simulink model "distortion_v4_1_saturation"  (R2018b)
settings: Solver=FixedStepDiscrete  StartTime=0.0  StopTime=(samples-1)/fs  RelTol=1e-3  EnableMultiTasking=on
InitFcn:
  | setup;
undefined symbols (not defined in the file): fs
libraries: dspvision x1
settings Model: Creator=ross  LastModifiedBy=eseny
settings DataIOCC: LimitDataPoints=on  SaveFormat=Array  SignalLogging=off
settings OptimizationCC: BlockReduction=off  ConditionallyExecuteInputs=off  DefaultParameterBehavior=Inlined  LifeSpan=inf
settings DebuggingCC: AlgebraicLoopMsg=error  UnderspecifiedInitializationDetection=Classic  MergeDetectMultiDrivingBlocksExec=none  SolverPrmCheckMsg=warning  Int32ToFloatConvMsg=none  StateNameClashWarn=warning  SFUnexpectedBacktrackingDiag=warning  SFNoUnconditionalDefaultTransitionDiag=warning  SFExecutionAtInitializationDiag=none
settings HardwareCC: ProdBitPerPointer=32  ProdBitPerSizeT=32  ProdBitPerPtrDiffT=32  ProdLargestAtomicFloat=None  ProdIntDivRoundTo=Undefined  ProdEndianess=Unspecified  ProdWordSize=32  ProdHWDeviceType=ASIC/FPGA->ASIC/FPGA  ProdEqTarget=off
settings ModelReferenceCC: PropagateSignalLabelsOutOfModel=off
settings SFSimCC: SimUseLocalCustomCode=off
settings RTWCC: RTWUseLocalCustomCode=off
settings CodeAppCC: StateflowObjectComments=on
settings GRTTargetCC: TargetLangStandard=C89/C90 (ANSI)  GeneratePreprocessorConditionals=Disable all
settings ConfigComp: CovMetricSettings=dw  CovHtmlReporting=on  CovSaveCumulativeToWorkspaceVar=on  CovSaveSingleToWorkspaceVar=on  CovExternalEMLEnable=off

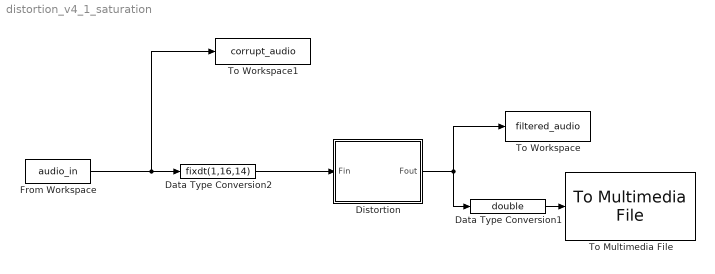
== system distortion_v4_1_saturation ==
  Data Type Conversion1 : DataTypeConversion  OutDataTypeStr=double
  Data Type Conversion2 : DataTypeConversion  OutDataTypeStr=fixdt(1,16,14)
  Distortion : Subsystem  TreatAsAtomicUnit=on
  From Workspace : FromWorkspace  VariableName=audio_in  SampleTime=1/fs  Interpolate=off  OutputAfterFinalValue=Holding final value
  To Multimedia File : dspvision/To Multimedia File  outputFilename=C:\Zynk_Book\hdl_reverb\distortion_audio.wav  streamSelection=Audio only  videoCompressor=None (uncompressed)  audioCompressor=None (uncompressed)  imagePorts=One multidimensional signal  fileType=WAV  audioDatatype=Determine from input data type  fourcc=RGB  videoQuality=75  mj2000CompFactor=10
      settings: SourceProductName=Computer Vision System Toolbox  SourceProductBaseCode=VP
  To Workspace : ToWorkspace  VariableName=filtered_audio  SampleTime=-1
  To Workspace1 : ToWorkspace  VariableName=corrupt_audio  SampleTime=-1
  wires:
  From Workspace/1 -> To Workspace1/1, Data Type Conversion2/1
  Distortion/1(Fout) -> To Workspace/1, Data Type Conversion1/1
  Data Type Conversion2/1 -> Distortion/1(Fin)
  Data Type Conversion1/1 -> To Multimedia File/1

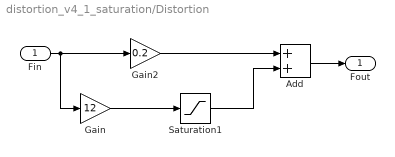
== system distortion_v4_1_saturation/Distortion ==
  Fin : Inport
  Add : Sum  OutDataTypeStr=fixdt(1,16,14)
  Gain : Gain  Gain=12  OutDataTypeStr=Inherit: Same as input
  Gain2 : Gain  Gain=0.2  OutDataTypeStr=Inherit: Same as input
  Saturation1 : Saturate  UpperLimit=0.05  LowerLimit=-0.05
  Fout : Outport
  wires:
  Fin/1 -> Gain2/1, Gain/1
  Gain/1 -> Saturation1/1
  Add/1 -> Fout/1
  Saturation1/1 -> Add/2
  Gain2/1 -> Add/1
